simulink subsystem "cut_and_shift"  (R2023b)
settings: Solver=VariableStepAuto  StartTime=0.0  StopTime=10.0  RelTol=1e-3
values from neighbouring files (symbols this model uses):
  fs = f_resample    [inizio.m]    (also in load_preset_audio.m; resample_workspace.m)
settings Model: Creator=Edp  LastModifiedBy=giorg

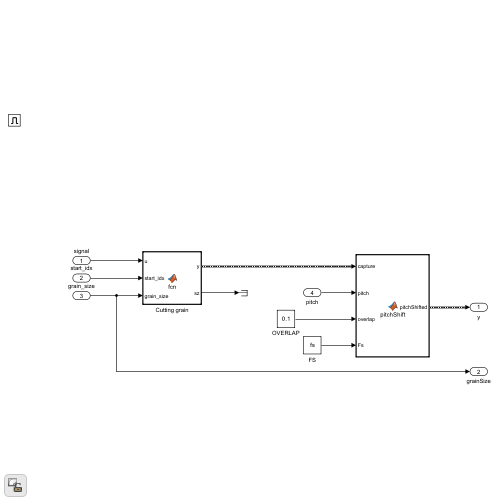
[thumbnail: Simulink's stored preview of the top-level diagram]
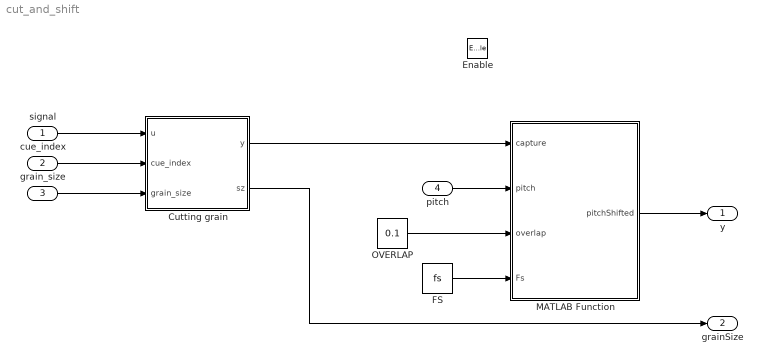
== system cut_and_shift ==
  signal : Inport
  cue_index : Inport  Port=2
  grain_size : Inport  Port=3
  pitch : Inport  Port=4
  Enable : EnablePort  PropagateVarSize=During execution
  Cutting grain : MATLAB Function  TreatAsAtomicUnit=on
  FS : Constant  Value=fs
  MATLAB Function : MATLAB Function  TreatAsAtomicUnit=on
  OVERLAP : Constant  Value=0.1
  y : Outport
  grainSize : Outport  Port=2
  wires:
  Cutting grain/2(sz) -> grainSize/1
  grain_size/1 -> Cutting grain/3(grain_size)
  Cutting grain/1(y) -> MATLAB Function/1(capture)
  signal/1 -> Cutting grain/1(u)
  pitch/1 -> MATLAB Function/2(pitch)
  MATLAB Function/1(pitchShifted) -> y/1
  OVERLAP/1 -> MATLAB Function/3(overlap)
  FS/1 -> MATLAB Function/4(Fs)
  cue_index/1 -> Cutting grain/2(cue_index)

== matlab function cut_and_shift/Cutting grain ==
  data: u input; y output size=120000; cue_index input; grain_size input; sz output
% INPUT: whole audio signal (u), starting point of the grain (cue_index),
% size of the grain(grain_size)

% OUTPUT: samples of the extracted grain (y), size of the grain (sz = grain_size) 
function [y, sz] = fcn(u, cue_index, grain_size)
end_idx = cue_index + grain_size;
y = u(cue_index:end_idx);
sz = size(y,1);

== matlab function cut_and_shift/MATLAB Function ==
  data: capture input; pitchShifted output size=120000; pitch input; overlap input; Fs input
function pitchShifted = pitchShift(capture, pitch, overlap, Fs)
%pitchShift Pitch shift algorithm 
% Copyrights 2018-2019 The MathWorks, Inc.

%#codegen
resetFlag = 0;      % Reset flag set to 0

persistent pitchShifter
if isempty(pitchShifter)
    pitchShifter = PitchShifter( ...
        'PitchShift',8,'Overlap',0.3);
    setSampleRate(pitchShifter,Fs);
end

pitchShifted = zeros(size(double(capture)),'like',double(capture));

if nargin > 4 && resetFlag
    reset(pitchShifter);
    return;
end

pitchShifter.PitchShift = pitch;
pitchShifter.Overlap = overlap;

[pitchShifted] = pitchShifter(double(capture));

end
